simulink library "calcTurnAngleInTangentFrame_ul"  (R2020a)
settings: Solver=VariableStepAuto  StartTime=0.0  StopTime=10.0  RelTol=1e-3
settings Model: Creator=Ayaz  LastModifiedBy=Ayaz

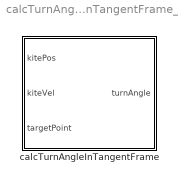
== system calcTurnAngleInTangentFrame_ul ==
  calcTurnAngleInTangentFrame : Subsystem

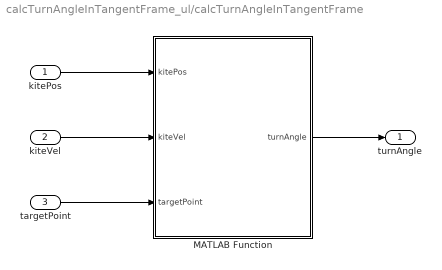
== system calcTurnAngleInTangentFrame_ul/calcTurnAngleInTangentFrame ==
  kitePos : Inport
  kiteVel : Inport  Port=2
  targetPoint : Inport  Port=3
  MATLAB Function : MATLAB Function  TreatAsAtomicUnit=on
  turnAngle : Outport
  wires:
  targetPoint/1 -> MATLAB Function/3(targetPoint)
  kiteVel/1 -> MATLAB Function/2(kiteVel)
  kitePos/1 -> MATLAB Function/1(kitePos)
  MATLAB Function/1(turnAngle) -> turnAngle/1

== matlab function calcTurnAngleInTangentFrame_ul/calcTurnAngleInTangentFrame/MATLAB Function ==
  data: kitePos input; turnAngle output; kiteVel input; targetPoint input
function turnAngle = calcTurnAngleInTangentFrame(kitePos,kiteVel,targetPoint)

turnAngle = calcTurnAngleInTangentFrame(kitePos,kiteVel,targetPoint);

end
